simulink model "Reverb_Setup_Pop"  (R2016b)
settings: Solver=VariableStepAuto  StartTime=0.0  StopTime=inf  RelTol=1e-3
libraries: simulink x10, dspvision x5, audioeffects x2, dspsnks4 x1
settings Model: Creator=Abhinav  LastModifiedBy=Abhinav

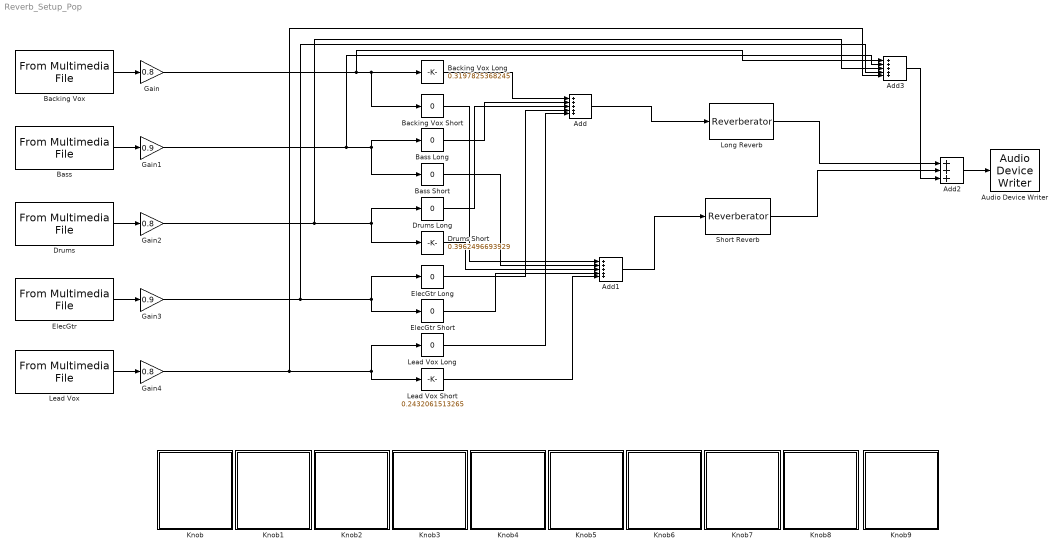
== system Reverb_Setup_Pop ==
  Add : Sum  Inputs=+++++
  Add1 : Sum  Inputs=+++++
  Add2 : Sum  Inputs=+++
  Add3 : Sum  Inputs=+++++
  Audio Device Writer : dspsnks4/Audio Device Writer  Driver=DirectSound  Device=Default  InheritSampleRate=on  SampleRate=44100  BitDepth=16-bit integer  BufferSize=4096  NumBuffers=10  DefaultOutputChannelMapping=on  OutputChannelMapping=1:2  OutputNumUnderrunSamples=off  DriverIdx=1  DeviceWarnFlag=''
  Backing Vox : dspvision/From Multimedia File  inputFilename=C:\Users\Abhinav\Desktop\Edited Excerpts\Audio_Files_Modified\Pop\Backing Vox Edited.wav  loop=on  numPlays=inf  outputStreams=Audio only  videoDataType=single  audioDataType=double  inheritSampleTime=on  userDefinedSampleTime=1/30  noAudioOutput=off  isIntensityVideo=off  fourcc=RGB  colorVideoFormat=Separate color signals  outputEOF=off  dataOrg=Column-major  audioFrameSize=4096  computeAudioFrameSize=off  outSamplingMode=Sample based
  Backing Vox Long : simulink/Math Operations/Slider Gain  low=0  gain=0.3197825368245  high=1
  Backing Vox Short : simulink/Math Operations/Slider Gain  low=0  gain=0  high=1
  Bass : dspvision/From Multimedia File  inputFilename=C:\Users\Abhinav\Desktop\Edited Excerpts\Audio_Files_Modified\Pop\Bass Edited.wav  loop=on  numPlays=inf  outputStreams=Audio only  videoDataType=single  audioDataType=double  inheritSampleTime=on  userDefinedSampleTime=1/30  noAudioOutput=off  isIntensityVideo=off  fourcc=RGB  colorVideoFormat=Separate color signals  outputEOF=off  dataOrg=Column-major  audioFrameSize=4096  computeAudioFrameSize=off  outSamplingMode=Sample based
  Bass Long : simulink/Math Operations/Slider Gain  low=0  gain=0  high=1
  Bass Short : simulink/Math Operations/Slider Gain  low=0  gain=0  high=1
  Drums : dspvision/From Multimedia File  inputFilename=C:\Users\Abhinav\Desktop\Edited Excerpts\Audio_Files_Modified\Pop\Drums Combined.wav  loop=on  numPlays=inf  outputStreams=Audio only  videoDataType=single  audioDataType=double  inheritSampleTime=on  userDefinedSampleTime=1/30  noAudioOutput=off  isIntensityVideo=off  fourcc=RGB  colorVideoFormat=Separate color signals  outputEOF=off  dataOrg=Column-major  audioFrameSize=4096  computeAudioFrameSize=off  outSamplingMode=Sample based
  Drums Long : simulink/Math Operations/Slider Gain  low=0  gain=0  high=1
  Drums Short : simulink/Math Operations/Slider Gain  low=0  gain=0.3962496693929  high=1
  ElecGtr : dspvision/From Multimedia File  inputFilename=C:\Users\Abhinav\Desktop\Edited Excerpts\Audio_Files_Modified\Pop\ElecGtr Edited.wav  loop=on  numPlays=inf  outputStreams=Audio only  videoDataType=single  audioDataType=double  inheritSampleTime=on  userDefinedSampleTime=1/30  noAudioOutput=off  isIntensityVideo=off  fourcc=RGB  colorVideoFormat=Separate color signals  outputEOF=off  dataOrg=Column-major  audioFrameSize=4096  computeAudioFrameSize=off  outSamplingMode=Sample based
  ElecGtr Long : simulink/Math Operations/Slider Gain  low=0  gain=0  high=1
  ElecGtr Short : simulink/Math Operations/Slider Gain  low=0  gain=0  high=1
  Gain : Gain  Gain=0.8
  Gain1 : Gain  Gain=0.9
  Gain2 : Gain  Gain=0.8
  Gain3 : Gain  Gain=0.9
  Gain4 : Gain  Gain=0.8
  Knob : Subsystem  DialogController=hmiCreateDDGDialog  IsWebBlock=on  mask(MWDashboardBlock){webBlockId=d1b1aeea-1a4c-4232-bc5c-ca080e2334c9, webBlockType=continuousknob, ShowInLibBrowser=on, ShowInitialText=on, HMISrcModelName=Reverb_Setup_Pop}
      mask prompts: webBlockId "WebBlock Id"; webBlockType "WebBlock Type"; HMISrcModelName "Source Model"
      mask help: SimulinkHMI:dialogs:ContinuousKnobDialogDesc
      mask Help: helpview([docroot '/mapfiles/simulink.map'], 'hmi_knob')
      mask Display:
      | if strcmp(get_param(bdroot(gcb),'BlockDiagramType'), 'library')
      |     image([(matlabroot) '/toolbox/simulink/hmi/icons/ContinuousKnob.png']);
      | end
  Knob1 : Subsystem  DialogController=hmiCreateDDGDialog  IsWebBlock=on  mask(MWDashboardBlock){webBlockId=eae3fb9e-6558-4900-a6d4-f6d46d805a51, webBlockType=continuousknob, ShowInLibBrowser=on, ShowInitialText=on, HMISrcModelName=Reverb_Setup_Pop}
      mask prompts: webBlockId "WebBlock Id"; webBlockType "WebBlock Type"; HMISrcModelName "Source Model"
      mask help: SimulinkHMI:dialogs:ContinuousKnobDialogDesc
      mask Help: helpview([docroot '/mapfiles/simulink.map'], 'hmi_knob')
      mask Display:
      | if strcmp(get_param(bdroot(gcb),'BlockDiagramType'), 'library')
      |     image([(matlabroot) '/toolbox/simulink/hmi/icons/ContinuousKnob.png']);
      | end
  Knob2 : Subsystem  DialogController=hmiCreateDDGDialog  IsWebBlock=on  mask(MWDashboardBlock){webBlockId=2ffb3fd0-a504-4a89-a812-3e52641839ce, webBlockType=continuousknob, ShowInLibBrowser=on, ShowInitialText=on, HMISrcModelName=Reverb_Setup_Pop}
      mask prompts: webBlockId "WebBlock Id"; webBlockType "WebBlock Type"; HMISrcModelName "Source Model"
      mask help: SimulinkHMI:dialogs:ContinuousKnobDialogDesc
      mask Help: helpview([docroot '/mapfiles/simulink.map'], 'hmi_knob')
      mask Display:
      | if strcmp(get_param(bdroot(gcb),'BlockDiagramType'), 'library')
      |     image([(matlabroot) '/toolbox/simulink/hmi/icons/ContinuousKnob.png']);
      | end
  Knob3 : Subsystem  DialogController=hmiCreateDDGDialog  IsWebBlock=on  mask(MWDashboardBlock){webBlockId=eff0b3fb-9bbf-432e-8a21-a781c492e988, webBlockType=continuousknob, ShowInLibBrowser=on, ShowInitialText=on, HMISrcModelName=Reverb_Setup_Pop}
      mask prompts: webBlockId "WebBlock Id"; webBlockType "WebBlock Type"; HMISrcModelName "Source Model"
      mask help: SimulinkHMI:dialogs:ContinuousKnobDialogDesc
      mask Help: helpview([docroot '/mapfiles/simulink.map'], 'hmi_knob')
      mask Display:
      | if strcmp(get_param(bdroot(gcb),'BlockDiagramType'), 'library')
      |     image([(matlabroot) '/toolbox/simulink/hmi/icons/ContinuousKnob.png']);
      | end
  Knob4 : Subsystem  DialogController=hmiCreateDDGDialog  IsWebBlock=on  mask(MWDashboardBlock){webBlockId=90b1255a-7ef6-498d-845b-50301710b1ab, webBlockType=continuousknob, ShowInLibBrowser=on, ShowInitialText=on, HMISrcModelName=Reverb_Setup_Pop}
      mask prompts: webBlockId "WebBlock Id"; webBlockType "WebBlock Type"; HMISrcModelName "Source Model"
      mask help: SimulinkHMI:dialogs:ContinuousKnobDialogDesc
      mask Help: helpview([docroot '/mapfiles/simulink.map'], 'hmi_knob')
      mask Display:
      | if strcmp(get_param(bdroot(gcb),'BlockDiagramType'), 'library')
      |     image([(matlabroot) '/toolbox/simulink/hmi/icons/ContinuousKnob.png']);
      | end
  Knob5 : Subsystem  DialogController=hmiCreateDDGDialog  IsWebBlock=on  mask(MWDashboardBlock){webBlockId=ce13f701-c396-43f0-b5e7-56cad611216b, webBlockType=continuousknob, ShowInLibBrowser=on, ShowInitialText=on, HMISrcModelName=Reverb_Setup_Pop}
      mask prompts: webBlockId "WebBlock Id"; webBlockType "WebBlock Type"; HMISrcModelName "Source Model"
      mask help: SimulinkHMI:dialogs:ContinuousKnobDialogDesc
      mask Help: helpview([docroot '/mapfiles/simulink.map'], 'hmi_knob')
      mask Display:
      | if strcmp(get_param(bdroot(gcb),'BlockDiagramType'), 'library')
      |     image([(matlabroot) '/toolbox/simulink/hmi/icons/ContinuousKnob.png']);
      | end
  Knob6 : Subsystem  DialogController=hmiCreateDDGDialog  IsWebBlock=on  mask(MWDashboardBlock){webBlockId=d3999bd8-71c9-4165-89f8-2401c53edfbd, webBlockType=continuousknob, ShowInLibBrowser=on, ShowInitialText=on, HMISrcModelName=Reverb_Setup_Pop}
      mask prompts: webBlockId "WebBlock Id"; webBlockType "WebBlock Type"; HMISrcModelName "Source Model"
      mask help: SimulinkHMI:dialogs:ContinuousKnobDialogDesc
      mask Help: helpview([docroot '/mapfiles/simulink.map'], 'hmi_knob')
      mask Display:
      | if strcmp(get_param(bdroot(gcb),'BlockDiagramType'), 'library')
      |     image([(matlabroot) '/toolbox/simulink/hmi/icons/ContinuousKnob.png']);
      | end
  Knob7 : Subsystem  DialogController=hmiCreateDDGDialog  IsWebBlock=on  mask(MWDashboardBlock){webBlockId=7fbba40c-88ce-4d7d-b793-d982e973495c, webBlockType=continuousknob, ShowInLibBrowser=on, ShowInitialText=on, HMISrcModelName=Reverb_Setup_Pop}
      mask prompts: webBlockId "WebBlock Id"; webBlockType "WebBlock Type"; HMISrcModelName "Source Model"
      mask help: SimulinkHMI:dialogs:ContinuousKnobDialogDesc
      mask Help: helpview([docroot '/mapfiles/simulink.map'], 'hmi_knob')
      mask Display:
      | if strcmp(get_param(bdroot(gcb),'BlockDiagramType'), 'library')
      |     image([(matlabroot) '/toolbox/simulink/hmi/icons/ContinuousKnob.png']);
      | end
  Knob8 : Subsystem  DialogController=hmiCreateDDGDialog  IsWebBlock=on  mask(MWDashboardBlock){webBlockId=dca59ee9-db92-495f-a509-51f10b6f0128, webBlockType=continuousknob, ShowInLibBrowser=on, ShowInitialText=on, HMISrcModelName=Reverb_Setup_Pop}
      mask prompts: webBlockId "WebBlock Id"; webBlockType "WebBlock Type"; HMISrcModelName "Source Model"
      mask help: SimulinkHMI:dialogs:ContinuousKnobDialogDesc
      mask Help: helpview([docroot '/mapfiles/simulink.map'], 'hmi_knob')
      mask Display:
      | if strcmp(get_param(bdroot(gcb),'BlockDiagramType'), 'library')
      |     image([(matlabroot) '/toolbox/simulink/hmi/icons/ContinuousKnob.png']);
      | end
  Knob9 : Subsystem  DialogController=hmiCreateDDGDialog  IsWebBlock=on  mask(MWDashboardBlock){webBlockId=e93f78a5-3240-4d52-91df-dd290e0cc59e, webBlockType=continuousknob, ShowInLibBrowser=on, ShowInitialText=on, HMISrcModelName=Reverb_Setup_Pop}
      mask prompts: webBlockId "WebBlock Id"; webBlockType "WebBlock Type"; HMISrcModelName "Source Model"
      mask help: SimulinkHMI:dialogs:ContinuousKnobDialogDesc
      mask Help: helpview([docroot '/mapfiles/simulink.map'], 'hmi_knob')
      mask Display:
      | if strcmp(get_param(bdroot(gcb),'BlockDiagramType'), 'library')
      |     image([(matlabroot) '/toolbox/simulink/hmi/icons/ContinuousKnob.png']);
      | end
  Lead Vox : dspvision/From Multimedia File  inputFilename=C:\Users\Abhinav\Desktop\Edited Excerpts\Audio_Files_Modified\Pop\Lead Vox Edited.wav  loop=on  numPlays=inf  outputStreams=Audio only  videoDataType=single  audioDataType=double  inheritSampleTime=on  userDefinedSampleTime=1/30  noAudioOutput=off  isIntensityVideo=off  fourcc=RGB  colorVideoFormat=Separate color signals  outputEOF=off  dataOrg=Column-major  audioFrameSize=4096  computeAudioFrameSize=off  outSamplingMode=Sample based
  Lead Vox Long : simulink/Math Operations/Slider Gain  low=0  gain=0  high=1
  Lead Vox Short : simulink/Math Operations/Slider Gain  low=0  gain=0.2432061513265  high=1
  Long Reverb : audioeffects/Reverberator  PreDelay=0.100  HighCutFrequency=20000  Diffusion=0.50  DecayFactor=0.20  HighFrequencyDamping=0.350  WetDryMix=1.000  InheritSampleRate=on  SampleRate=44100  SimulateUsing=Interpreted execution
  Short Reverb : audioeffects/Reverberator  PreDelay=0.010  HighCutFrequency=20000  Diffusion=0.50  DecayFactor=0.800  HighFrequencyDamping=0.450  WetDryMix=1.000  InheritSampleRate=on  SampleRate=44100  SimulateUsing=Interpreted execution
  wires:
  Backing Vox/1 -> Gain/1
  Bass/1 -> Gain1/1
  Drums/1 -> Gain2/1
  ElecGtr/1 -> Gain3/1
  Lead Vox/1 -> Gain4/1
  Backing Vox Long/1 -> Add/1
  Bass Long/1 -> Add/2
  Drums Long/1 -> Add/3
  ElecGtr Long/1 -> Add/4
  Lead Vox Long/1 -> Add/5
  Backing Vox Short/1 -> Add1/1
  Bass Short/1 -> Add1/2
  Drums Short/1 -> Add1/3
  ElecGtr Short/1 -> Add1/4
  Lead Vox Short/1 -> Add1/5
  Add/1 -> Long Reverb/1
  Add1/1 -> Short Reverb/1
  Long Reverb/1 -> Add2/1
  Short Reverb/1 -> Add2/2
  Add2/1 -> Audio Device Writer/1
  Gain/1 -> Add3/1, Backing Vox Short/1, Backing Vox Long/1
  Gain1/1 -> Add3/2, Bass Short/1, Bass Long/1
  Gain2/1 -> Add3/3, Drums Long/1, Drums Short/1
  Gain3/1 -> Add3/4, ElecGtr Long/1, ElecGtr Short/1
  Gain4/1 -> Add3/5, Lead Vox Long/1, Lead Vox Short/1
  Add3/1 -> Add2/3

== system Reverb_Setup_Pop/Knob ==

== system Reverb_Setup_Pop/Knob1 ==

== system Reverb_Setup_Pop/Knob2 ==

== system Reverb_Setup_Pop/Knob3 ==

== system Reverb_Setup_Pop/Knob4 ==

== system Reverb_Setup_Pop/Knob5 ==

== system Reverb_Setup_Pop/Knob6 ==

== system Reverb_Setup_Pop/Knob7 ==

== system Reverb_Setup_Pop/Knob8 ==

== system Reverb_Setup_Pop/Knob9 ==
